simulink model "compswitchA"  (R2025a)
settings: Solver=VariableStepAuto  StartTime=0.0  StopTime=10.0  RelTol=1e-3
libraries: StdLib x8, PaperLib x2
settings Model: Creator=peter  LastModifiedBy=peter
settings RTWCC: GPUComputeCapability=3.5

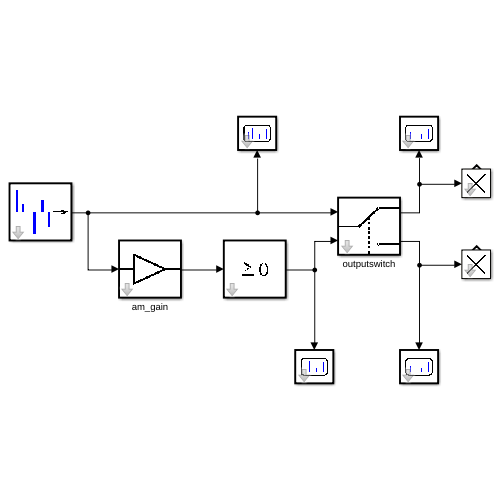
[thumbnail: Simulink's stored preview of the top-level diagram]
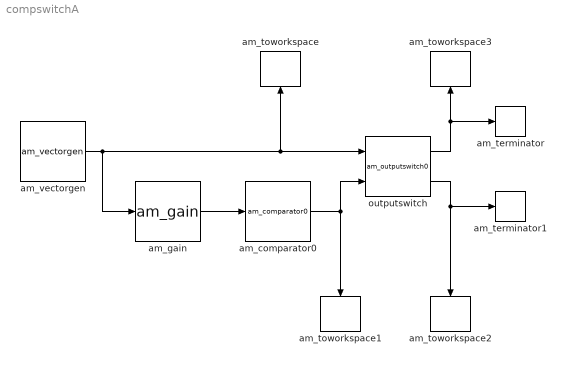
== system compswitchA ==
  am_comparator0 : PaperLib/am_comparator0  tau=[0,1]  debug=0
  am_gain : StdLib/am_gain  g=1  tau=[0,1]  debug=0
      settings: SourceProductName=Math Operations
  am_terminator : StdLib/am_terminator  tau=[0,1]  debug=0
  am_terminator1 : StdLib/am_terminator  tau=[0,1]  debug=0
  am_toworkspace : StdLib/am_toworkspace  varname="\"vgenOut\""  t0=0  format="\"vector\""  tau=[0,5]  debug=0
  am_toworkspace1 : StdLib/am_toworkspace  varname="\"compOut\""  t0=0  format="\"vector\""  tau=[0,5]  debug=0
  am_toworkspace2 : StdLib/am_toworkspace  varname="\"sw2Out\""  t0=0  format="\"vector\""  tau=[0,5]  debug=0
  am_toworkspace3 : StdLib/am_toworkspace  varname="\"sw1Out\""  t0=0  format="\"vector\""  tau=[0,5]  debug=0
  am_vectorgen : StdLib/am_vectorgen  tvec=[1, 3, 7, 8, 9]  yvec=[2, -3, -2, 1, -1]  tau=[0,1]  debug=0
  outputswitch : PaperLib/am_outputswitch0  port0=1  tau=[0,2]  debug=0
      settings: SourceProductName=Routing
  wires:
  am_vectorgen/1 -> am_gain/1, am_toworkspace/1, outputswitch/1
  outputswitch/1 -> am_toworkspace3/1, am_terminator/1
  outputswitch/2 -> am_toworkspace2/1, am_terminator1/1
  am_comparator0/1 -> am_toworkspace1/1, outputswitch/2
  am_gain/1 -> am_comparator0/1
